simulink library "NREL5MW_Library"  (Simulink 8.2)
settings: Solver=ode45  StartTime=0.0  StopTime=10.0  RelTol=1e-3
undefined symbols (not defined in the file): NDOF, NumOuts, OutList, Parameter, q_init, qdot_init, strmatch, x1_t0
libraries: NREL5MW_Library x6, simulink x1
settings Model: Creator=raach  LastModifiedBy=schlipf

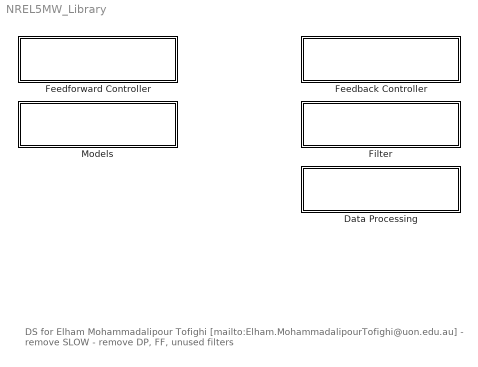
== system NREL5MW_Library ==
  note: DS for Elham Mohammadalipour Tofighi [mailto:Elham.MohammadalipourTofighi@uon.edu.au]
      | - remove SLOW
      | - remove DP, FF, unused filters
  Data Processing : Subsystem
      mask Display: fprintf('Data Processing')
  Feedback Controller : Subsystem
      mask Display: disp('Feedback Controller')
  Feedforward Controller : Subsystem
      mask Display: disp('Feedforward Controller')
  Filter : Subsystem
      mask Display: fprintf('Filter')
  Models : Subsystem
      mask Display: disp('Models')

== system NREL5MW_Library/Data Processing ==

== system NREL5MW_Library/Feedback Controller ==
  Feedback Controller : Subsystem
  Pitch Controller : Subsystem
  Torque Controller : Subsystem

== system NREL5MW_Library/Feedforward Controller ==

== system NREL5MW_Library/Filter ==
  FilterGenSpeed : Subsystem
  FilterSwitchR3 : Subsystem

== system NREL5MW_Library/Models ==
  FAST : Subsystem
  Generator : Subsystem
  Pitch Actuator : Subsystem

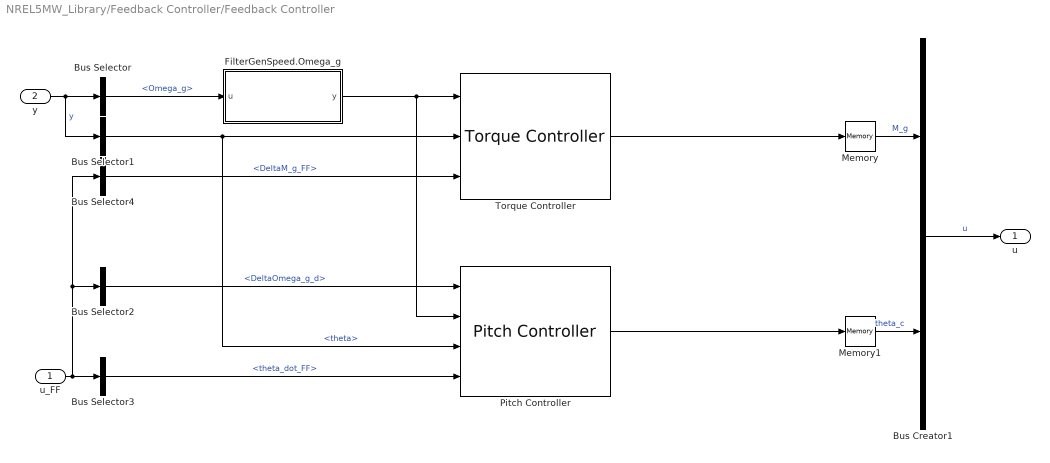
== system NREL5MW_Library/Feedback Controller/Feedback Controller ==
  u_FF : Inport
  y : Inport  Port=2
  Bus Creator1 : BusCreator  Inputs=2
  Bus Selector : BusSelector  OutputSignals=Omega_g
  Bus Selector1 : BusSelector  OutputSignals=theta
  Bus Selector2 : BusSelector  OutputSignals=DeltaOmega_g_d
  Bus Selector3 : BusSelector  OutputSignals=theta_dot_FF
  Bus Selector4 : BusSelector  OutputSignals=DeltaM_g_FF
  FilterGenSpeed.Omega_g : Subsystem
  Memory : Memory  X0=[Parameter.IC.M_g]
  Memory1 : Memory  X0=[Parameter.IC.theta]
  Pitch Controller : NREL5MW_Library/Feedback Controller/Pitch Controller
  Torque Controller : NREL5MW_Library/Feedback Controller/Torque Controller
  u : Outport
  wires:
  Bus Selector2/1 -> Pitch Controller/1  "<DeltaOmega_g_d>"
  Bus Selector/1 -> FilterGenSpeed.Omega_g/1(u)  "<Omega_g>"
  Bus Selector3/1 -> Pitch Controller/4  "<theta_dot_FF>"
  u_FF/1 -> Bus Selector3/1, Bus Selector4/1, Bus Selector2/1
  Pitch Controller/1 -> Memory1/1
  Bus Creator1/1 -> u/1  "u"
  Memory1/1 -> Bus Creator1/2  "theta_c"
  Memory/1 -> Bus Creator1/1  "M_g"
  Bus Selector1/1 -> Pitch Controller/3, Torque Controller/2  "<theta>"
  FilterGenSpeed.Omega_g/1(y) -> Torque Controller/1, Pitch Controller/2
  Torque Controller/1 -> Memory/1
  y/1 -> Bus Selector/1, Bus Selector1/1  "y"
  Bus Selector4/1 -> Torque Controller/3  "<DeltaM_g_FF>"

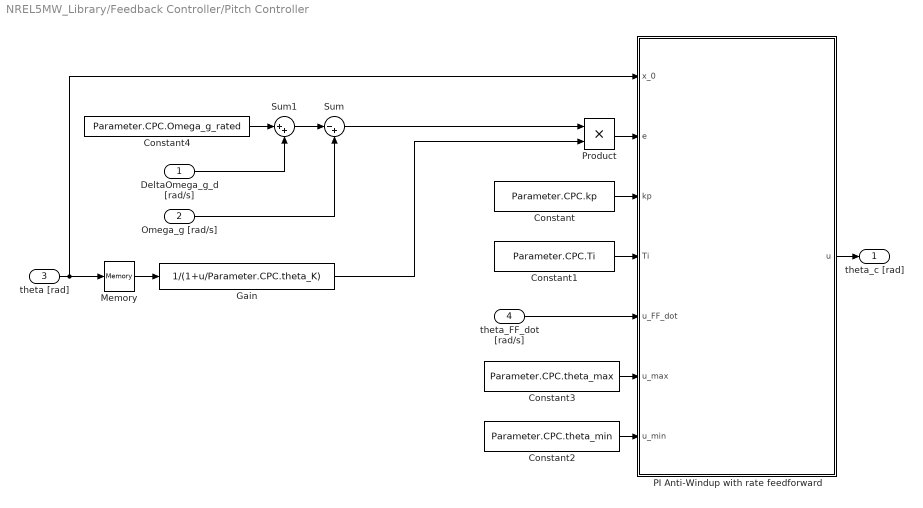
== system NREL5MW_Library/Feedback Controller/Pitch Controller ==
  DeltaOmega_g_d [rad/s] : Inport
  Omega_g [rad/s] : Inport  Port=2
  theta [rad] : Inport  Port=3
  theta_FF_dot [rad/s] : Inport  Port=4
  Constant : Constant  Value=Parameter.CPC.kp
  Constant1 : Constant  Value=Parameter.CPC.Ti
  Constant2 : Constant  Value=Parameter.CPC.theta_min
  Constant3 : Constant  Value=Parameter.CPC.theta_max
  Constant4 : Constant  Value=Parameter.CPC.Omega_g_rated
  Gain : Fcn  Expr=1/(1+u/Parameter.CPC.theta_K)
  Memory : Memory  X0=Parameter.IC.theta
  PI Anti-Windup with rate feedforward : Subsystem
  Product : Product  RndMeth=Zero
  Sum : Sum  Inputs=|-+
  Sum1 : Sum  Inputs=|++
  theta_c [rad] : Outport
  wires:
  Memory/1 -> Gain/1
  theta [rad]/1 -> PI Anti-Windup with rate feedforward/1(x_0), Memory/1
  Omega_g [rad/s]/1 -> Sum/2
  Gain/1 -> Product/2
  Sum/1 -> Product/1
  Product/1 -> PI Anti-Windup with rate feedforward/2(e)
  theta_FF_dot [rad/s]/1 -> PI Anti-Windup with rate feedforward/5(u_FF_dot)
  PI Anti-Windup with rate feedforward/1(u) -> theta_c [rad]/1
  Constant/1 -> PI Anti-Windup with rate feedforward/3(kp)
  Constant1/1 -> PI Anti-Windup with rate feedforward/4(Ti)
  Constant2/1 -> PI Anti-Windup with rate feedforward/7(u_min)
  Constant3/1 -> PI Anti-Windup with rate feedforward/6(u_max)
  DeltaOmega_g_d [rad/s]/1 -> Sum1/2
  Sum1/1 -> Sum/1
  Constant4/1 -> Sum1/1

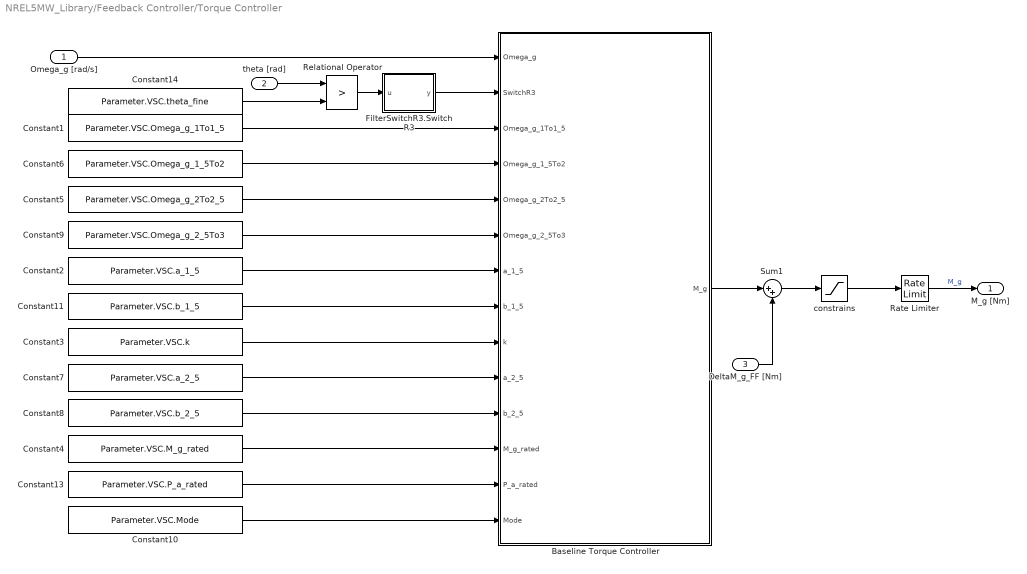
== system NREL5MW_Library/Feedback Controller/Torque Controller ==
  Omega_g [rad/s] : Inport
  theta [rad] : Inport  Port=2
  DeltaM_g_FF [Nm] : Inport  Port=3
  Baseline Torque Controller : MATLAB Function  TreatAsAtomicUnit=on
  Constant1 : Constant  Value=Parameter.VSC.Omega_g_1To1_5
  Constant10 : Constant  Value=Parameter.VSC.Mode
  Constant11 : Constant  Value=Parameter.VSC.b_1_5
  Constant13 : Constant  Value=Parameter.VSC.P_a_rated
  Constant14 : Constant  Value=Parameter.VSC.theta_fine
  Constant2 : Constant  Value=Parameter.VSC.a_1_5
  Constant3 : Constant  Value=Parameter.VSC.k
  Constant4 : Constant  Value=Parameter.VSC.M_g_rated
  Constant5 : Constant  Value=Parameter.VSC.Omega_g_2To2_5
  Constant6 : Constant  Value=Parameter.VSC.Omega_g_1_5To2
  Constant7 : Constant  Value=Parameter.VSC.a_2_5
  Constant8 : Constant  Value=Parameter.VSC.b_2_5
  Constant9 : Constant  Value=Parameter.VSC.Omega_g_2_5To3
  FilterSwitchR3.SwitchR3 : Subsystem
  Rate Limiter : RateLimiter  RisingSlewLimit=Parameter.VSC.M_g_dot_max  FallingSlewLimit=-Parameter.VSC.M_g_dot_max  SampleTimeMode=inherited  InitialCondition=Parameter.IC.M_g
  Relational Operator : RelationalOperator  Operator=>  OutDataTypeStr=boolean
  Sum1 : Sum  Inputs=|++
  constrains : Saturate  UpperLimit=Parameter.VSC.M_g_max  LowerLimit=Parameter.VSC.M_g_min
  M_g [Nm] : Outport
  wires:
  constrains/1 -> Rate Limiter/1
  Constant13/1 -> Baseline Torque Controller/13(P_a_rated)
  Constant11/1 -> Baseline Torque Controller/8(b_1_5)
  Constant2/1 -> Baseline Torque Controller/7(a_1_5)
  Constant10/1 -> Baseline Torque Controller/14(Mode)
  Constant3/1 -> Baseline Torque Controller/9(k)
  Constant7/1 -> Baseline Torque Controller/10(a_2_5)
  Constant8/1 -> Baseline Torque Controller/11(b_2_5)
  Constant4/1 -> Baseline Torque Controller/12(M_g_rated)
  Constant9/1 -> Baseline Torque Controller/6(Omega_g_2_5To3)
  Constant6/1 -> Baseline Torque Controller/4(Omega_g_1_5To2)
  Constant5/1 -> Baseline Torque Controller/5(Omega_g_2To2_5)
  Constant1/1 -> Baseline Torque Controller/3(Omega_g_1To1_5)
  Rate Limiter/1 -> M_g [Nm]/1  "M_g"
  Omega_g [rad/s]/1 -> Baseline Torque Controller/1(Omega_g)
  Baseline Torque Controller/1(M_g) -> Sum1/1
  Sum1/1 -> constrains/1
  DeltaM_g_FF [Nm]/1 -> Sum1/2
  Constant14/1 -> Relational Operator/2
  Relational Operator/1 -> FilterSwitchR3.SwitchR3/1(u)
  theta [rad]/1 -> Relational Operator/1
  FilterSwitchR3.SwitchR3/1(y) -> Baseline Torque Controller/2(SwitchR3)

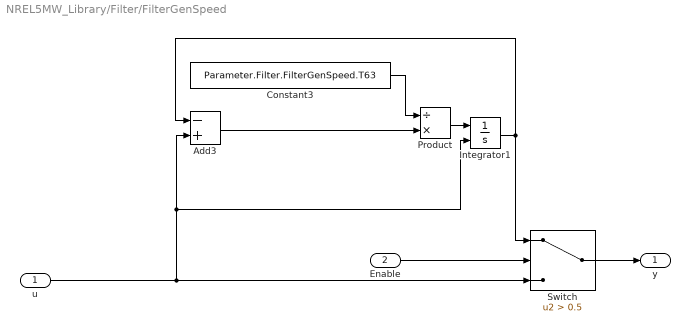
== system NREL5MW_Library/Filter/FilterGenSpeed ==
  u : Inport
  Enable : Inport  Port=2
  Add3 : Sum  Inputs=-+
  Constant3 : Constant  Value=Parameter.Filter.FilterGenSpeed.T63
  Integrator1 : Integrator  InitialConditionSource=external  InitialCondition=x1_t0
  Product : Product  Inputs=/*  RndMeth=Zero
  Switch : Switch  Criteria=u2 > Threshold  Threshold=0.5
  y : Outport
  wires:
  Constant3/1 -> Product/1
  Integrator1/1 -> Add3/1, Switch/1
  Product/1 -> Integrator1/1
  Add3/1 -> Product/2
  u/1 -> Switch/3, Integrator1/2, Add3/2
  Switch/1 -> y/1
  Enable/1 -> Switch/2

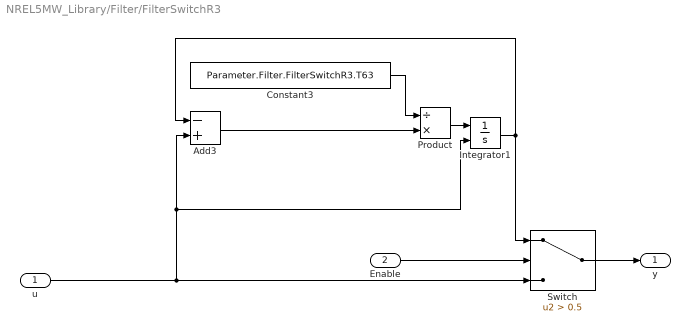
== system NREL5MW_Library/Filter/FilterSwitchR3 ==
  u : Inport
  Enable : Inport  Port=2
  Add3 : Sum  Inputs=-+
  Constant3 : Constant  Value=Parameter.Filter.FilterSwitchR3.T63
  Integrator1 : Integrator  InitialConditionSource=external  InitialCondition=x1_t0
  Product : Product  Inputs=/*  RndMeth=Zero
  Switch : Switch  Criteria=u2 > Threshold  Threshold=0.5
  y : Outport
  wires:
  Enable/1 -> Switch/2
  Switch/1 -> y/1
  u/1 -> Add3/2, Integrator1/2, Switch/3
  Add3/1 -> Product/2
  Product/1 -> Integrator1/1
  Integrator1/1 -> Switch/1, Add3/1
  Constant3/1 -> Product/1

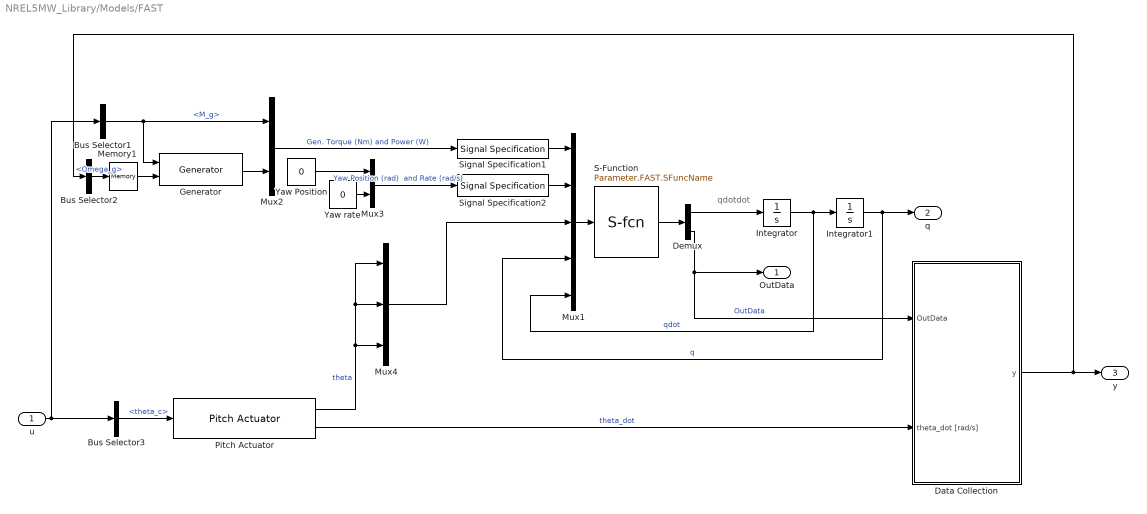
== system NREL5MW_Library/Models/FAST ==
  note: qdotdot
  u : Inport
  Bus Selector1 : BusSelector  OutputSignals=M_g
  Bus Selector2 : BusSelector  OutputSignals=Omega_g
  Bus Selector3 : BusSelector  OutputSignals=theta_c
  Data Collection : Subsystem
  Demux : Demux  Outputs=[NDOF, NumOuts]
  Generator : NREL5MW_Library/Models/Generator
  Integrator : Integrator  InitialCondition=qdot_init
  Integrator1 : Integrator  InitialCondition=q_init
  Memory1 : Memory  X0=Parameter.IC.Omega_g
  Mux1 : Mux  Inputs=5
  Mux2 : Mux  Inputs=2
  Mux3 : Mux  Inputs=2
  Mux4 : Mux  Inputs=3
  Pitch Actuator : NREL5MW_Library/Models/Pitch Actuator
  S-Function : S-Function  FunctionName=Parameter.FAST.SFuncName  EnableBusSupport=off
  Signal Specification1 : SignalSpecification  OutDataTypeStr=double  Dimensions=2
  Signal Specification2 : SignalSpecification  OutDataTypeStr=double  Dimensions=2
  Yaw Position : Constant  Value=0
  Yaw rate : Constant  Value=0
  OutData : Outport
  q : Outport  Port=2
  y : Outport  Port=3
  wires:
  Bus Selector1/1 -> Mux2/1, Generator/1  "<M_g>"
  Bus Selector3/1 -> Pitch Actuator/1  "<theta_c>"
  Pitch Actuator/2 -> Data Collection/2(theta_dot [rad/s])  "theta_dot"
  Mux4/1 -> Mux1/3
  u/1 -> Bus Selector3/1, Bus Selector1/1
  Integrator/1 -> Integrator1/1, Mux1/5  "qdot"
  Mux2/1 -> Signal Specification1/1  "Gen. Torque (Nm) and Power (W)"
  S-Function/1 -> Demux/1
  Demux/1 -> Integrator/1
  Demux/2 -> Data Collection/1(OutData), OutData/1  "OutData"
  Mux1/1 -> S-Function/1
  Mux3/1 -> Signal Specification2/1  "Yaw Position (rad)  and Rate (rad/s)"
  Integrator1/1 -> q/1, Mux1/4  "q"
  Signal Specification1/1 -> Mux1/1
  Signal Specification2/1 -> Mux1/2
  Yaw Position/1 -> Mux3/1
  Yaw rate/1 -> Mux3/2
  Pitch Actuator/1 -> Mux4/3, Mux4/1, Mux4/2  "theta"
  Data Collection/1(y) -> y/1, Bus Selector2/1
  Memory1/1 -> Generator/2
  Bus Selector2/1 -> Memory1/1  "<Omega_g>"
  Generator/1 -> Mux2/2

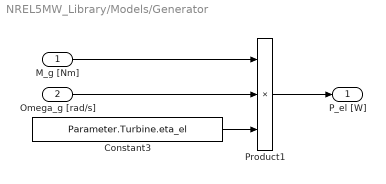
== system NREL5MW_Library/Models/Generator ==
  M_g [Nm] : Inport
  Omega_g [rad/s] : Inport  Port=2
  Constant3 : Constant  Value=Parameter.Turbine.eta_el
  Product1 : Product  Inputs=***  RndMeth=Zero
  P_el [W] : Outport
  wires:
  Constant3/1 -> Product1/3
  M_g [Nm]/1 -> Product1/1
  Product1/1 -> P_el [W]/1
  Omega_g [rad/s]/1 -> Product1/2

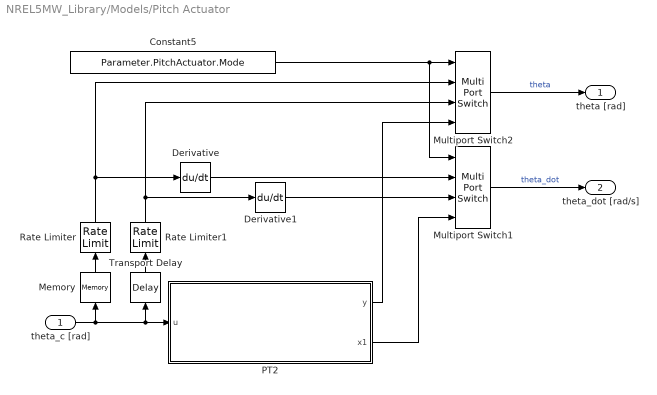
== system NREL5MW_Library/Models/Pitch Actuator ==
  theta_c [rad] : Inport
  Constant5 : Constant  Value=Parameter.PitchActuator.Mode
  Derivative : Derivative
  Derivative1 : Derivative
  Memory : Memory  X0=Parameter.IC.theta
  Multiport Switch1 : MultiPortSwitch  DataPortOrder=Specify indices  DataPortIndices={0,1,2}
  Multiport Switch2 : MultiPortSwitch  DataPortOrder=Specify indices  DataPortIndices={0,1,2}
  PT2 : Subsystem  mask{omega=Parameter.PitchActuator.omega, xi=Parameter.PitchActuator.xi, x1_t0=0, x2_t0=Parameter.IC.theta, x1_con=Parameter.PitchActuator.theta_dot_max, x2_max=Parameter.PitchActuator.theta_max, x2_min=Parameter.PitchActuator.theta_min}
      mask prompts: omega "undamped natural frequency [rad/s]"; xi "damping factor [-]"; x1_t0 "Inicial condition first state"; x2_t0 "Inicial condition second state"; x1_con "Constraint on first state (abs(x1)<=x1_con)"; x2_max "Upper bound x2"; x2_min "Lower bound x2"
      mask Display:
      | disp(['omega = ',num2str(omega),'\n'...
      |     ,'xi = ',num2str(xi),'\n'...
      |     ,'x1(t0) = ',num2str(x1_t0),'\n'...
      |     ,'x2(t0) = ',num2str(x2_t0),'\n'...
      |     ,'abs(x1) <= ',num2str(x1_con)])
      | port_label('output',1,'y')
      | port_label('output',2,'x1')
      | port_label('input',1,'u')
  Rate Limiter : RateLimiter  RisingSlewLimit=Parameter.PitchActuator.theta_dot_max  FallingSlewLimit=-Parameter.PitchActuator.theta_dot_max  SampleTimeMode=inherited  InitialCondition=Parameter.IC.theta
  Rate Limiter1 : RateLimiter  RisingSlewLimit=Parameter.PitchActuator.theta_dot_max  FallingSlewLimit=-Parameter.PitchActuator.theta_dot_max  SampleTimeMode=inherited  InitialCondition=Parameter.IC.theta
  Transport Delay : TransportDelay  DelayTime=Parameter.PitchActuator.Delay  InitialOutput=Parameter.IC.theta
  theta [rad] : Outport
  theta_dot [rad/s] : Outport  Port=2
  wires:
  Memory/1 -> Rate Limiter/1
  Rate Limiter/1 -> Multiport Switch2/2, Derivative/1
  Multiport Switch1/1 -> theta_dot [rad/s]/1  "theta_dot"
  Derivative/1 -> Multiport Switch1/2
  Multiport Switch2/1 -> theta [rad]/1  "theta"
  theta_c [rad]/1 -> Memory/1, Transport Delay/1, PT2/1(u)
  Constant5/1 -> Multiport Switch1/1, Multiport Switch2/1
  PT2/1(y) -> Multiport Switch2/4
  PT2/2(x1) -> Multiport Switch1/4
  Derivative1/1 -> Multiport Switch1/3
  Transport Delay/1 -> Rate Limiter1/1
  Rate Limiter1/1 -> Derivative1/1, Multiport Switch2/3

== system NREL5MW_Library/Feedback Controller/Feedback Controller/FilterGenSpeed.Omega_g ==
  u : Inport
  Constant3 : Constant  Value=Parameter.Filter.FilterGenSpeed.Omega_g.Enable
  FilterGenSpeed : NREL5MW_Library/Filter/FilterGenSpeed
  y : Outport
  wires:
  FilterGenSpeed/1 -> y/1
  u/1 -> FilterGenSpeed/1
  Constant3/1 -> FilterGenSpeed/2

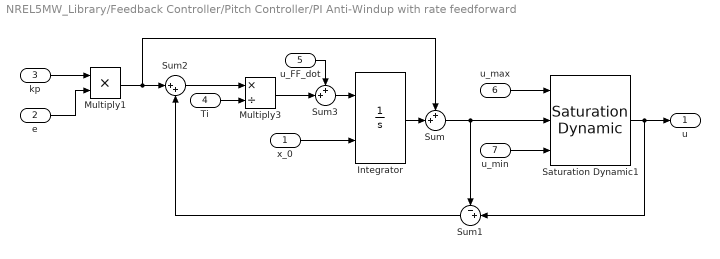
== system NREL5MW_Library/Feedback Controller/Pitch Controller/PI Anti-Windup with rate feedforward ==
  x_0 : Inport
  e : Inport  Port=2
  kp : Inport  Port=3
  Ti : Inport  Port=4
  u_FF_dot : Inport  Port=5
  u_max : Inport  Port=6
  u_min : Inport  Port=7
  Integrator : Integrator  InitialConditionSource=external
  Multiply1 : Product  Inputs=**
  Multiply3 : Product  Inputs=*/
  Saturation Dynamic1 : simulink/Discontinuities/Saturation Dynamic  OutMin=[]  OutMax=[]  OutDataTypeStr=Inherit: Same as second input  OutDataType=fixdt(1, 16)  OutScaling=2^-10  DoSatur=off
  Sum : Sum  Inputs=++|
  Sum1 : Sum  Inputs=-+|
  Sum2 : Sum  Inputs=|++
  Sum3 : Sum  Inputs=++|
  u : Outport
  wires:
  Saturation Dynamic1/1 -> u/1, Sum1/2
  Integrator/1 -> Sum/2
  kp/1 -> Multiply1/1
  e/1 -> Multiply1/2
  Ti/1 -> Multiply3/2
  Sum1/1 -> Sum2/2
  Multiply1/1 -> Sum/1, Sum2/1
  Sum2/1 -> Multiply3/1
  x_0/1 -> Integrator/2
  Multiply3/1 -> Sum3/2
  Sum3/1 -> Integrator/1
  u_FF_dot/1 -> Sum3/1
  u_min/1 -> Saturation Dynamic1/3
  Sum/1 -> Saturation Dynamic1/2, Sum1/1
  u_max/1 -> Saturation Dynamic1/1

== system NREL5MW_Library/Feedback Controller/Torque Controller/FilterSwitchR3.SwitchR3 ==
  u : Inport
  Constant3 : Constant  Value=Parameter.Filter.FilterSwitchR3.SwitchR3.Enable
  Data Type Conversion : DataTypeConversion  OutDataTypeStr=double
  FilterSwitchR3 : NREL5MW_Library/Filter/FilterSwitchR3
  y : Outport
  wires:
  Constant3/1 -> FilterSwitchR3/2
  u/1 -> Data Type Conversion/1
  FilterSwitchR3/1 -> y/1
  Data Type Conversion/1 -> FilterSwitchR3/1

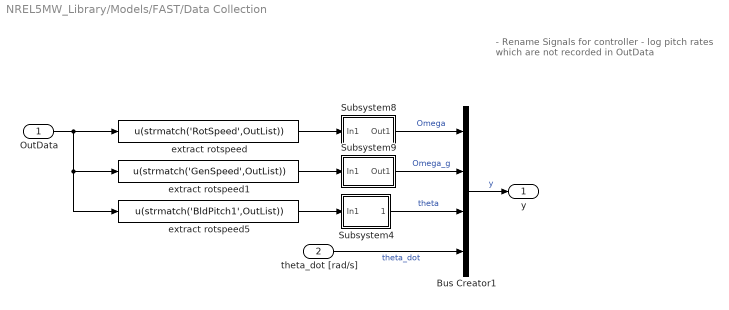
== system NREL5MW_Library/Models/FAST/Data Collection ==
  note: - Rename Signals for controller
      | - log pitch rates which are not recorded in OutData
  OutData : Inport
  theta_dot [rad/s] : Inport  Port=2
  Bus Creator1 : BusCreator
  Subsystem4 : Subsystem
      mask Display: disp('deg2rad')
  Subsystem8 : Subsystem
      mask Display: disp('rpm2rad/s')
  Subsystem9 : Subsystem
      mask Display: disp('rpm2rad/s')
  extract rotspeed : Fcn  Expr=u(strmatch('RotSpeed',OutList))
  extract rotspeed1 : Fcn  Expr=u(strmatch('GenSpeed',OutList))
  extract rotspeed5 : Fcn  Expr=u(strmatch('BldPitch1',OutList))
  y : Outport
  wires:
  Subsystem9/1(Out1) -> Bus Creator1/2  "Omega_g"
  Subsystem8/1(Out1) -> Bus Creator1/1  "Omega"
  extract rotspeed5/1 -> Subsystem4/1(In1)
  Bus Creator1/1 -> y/1  "y"
  extract rotspeed1/1 -> Subsystem9/1(In1)
  extract rotspeed/1 -> Subsystem8/1(In1)
  OutData/1 -> extract rotspeed1/1, extract rotspeed5/1, extract rotspeed/1
  Subsystem4/1(Out1) -> Bus Creator1/3  "theta"
  theta_dot [rad/s]/1 -> Bus Creator1/4  "theta_dot"

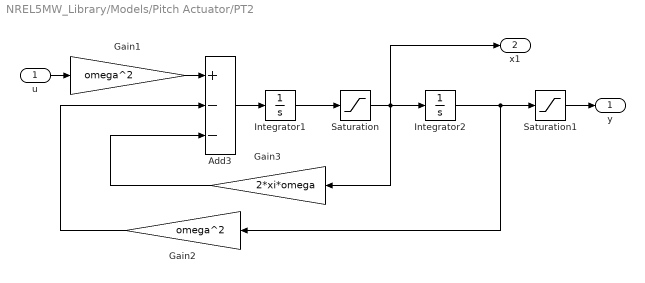
== system NREL5MW_Library/Models/Pitch Actuator/PT2 ==
  u : Inport
  Add3 : Sum  Inputs=+--
  Gain1 : Gain  Gain=omega^2  SaturateOnIntegerOverflow=on  OutDataTypeStr=Inherit: Same as input  ParamDataTypeStr=Inherit: Same as input
  Gain2 : Gain  Gain=omega^2  SaturateOnIntegerOverflow=on  OutDataTypeStr=Inherit: Same as input  ParamDataTypeStr=Inherit: Same as input
  Gain3 : Gain  Gain=2*xi*omega  SaturateOnIntegerOverflow=on  OutDataTypeStr=Inherit: Same as input  ParamDataTypeStr=Inherit: Same as input
  Integrator1 : Integrator  InitialCondition=x1_t0
  Integrator2 : Integrator  InitialCondition=x2_t0
  Saturation : Saturate  UpperLimit=x1_con  LowerLimit=-x1_con
  Saturation1 : Saturate  UpperLimit=x2_max  LowerLimit=x2_min
  y : Outport
  x1 : Outport  Port=2
  wires:
  Saturation1/1 -> y/1
  Gain3/1 -> Add3/3
  Integrator2/1 -> Saturation1/1, Gain2/1
  Integrator1/1 -> Saturation/1
  u/1 -> Gain1/1
  Add3/1 -> Integrator1/1
  Gain1/1 -> Add3/1
  Gain2/1 -> Add3/2
  Saturation/1 -> x1/1, Gain3/1, Integrator2/1

== system NREL5MW_Library/Models/FAST/Data Collection/Subsystem4 ==
  In1 : Inport
  deg in rad : Gain  Gain=2*pi/360  SaturateOnIntegerOverflow=on  OutDataTypeStr=Inherit: Same as input  ParamDataTypeStr=Inherit: Same as input
  Out1 : Outport
  wires:
  In1/1 -> deg in rad/1
  deg in rad/1 -> Out1/1

== system NREL5MW_Library/Models/FAST/Data Collection/Subsystem8 ==
  In1 : Inport
  rpm in rad/s : Gain  Gain=2*pi/60  SaturateOnIntegerOverflow=on  OutDataTypeStr=Inherit: Same as input  ParamDataTypeStr=Inherit: Same as input
  Out1 : Outport
  wires:
  rpm in rad/s/1 -> Out1/1
  In1/1 -> rpm in rad/s/1

== system NREL5MW_Library/Models/FAST/Data Collection/Subsystem9 ==
  In1 : Inport
  rpm in rad/s : Gain  Gain=2*pi/60  SaturateOnIntegerOverflow=on  OutDataTypeStr=Inherit: Same as input  ParamDataTypeStr=Inherit: Same as input
  Out1 : Outport
  wires:
  In1/1 -> rpm in rad/s/1
  rpm in rad/s/1 -> Out1/1

== matlab function Feedback Controller/Torque Controller/Baseline Torque Controller ==
  settings: fimath=|
      | fimath(...
      | 'RoundMode', 'floor',...
      | 'OverflowMode', 'wrap',...
      | 'ProductMode', 'KeepLSB', 'ProductWordLength', 32,...
      | 'SumMode', 'KeepLSB', 'SumWordLength', 32,...
      | 'CastBeforeSum', false)
  data: Omega_g input double; SwitchR3 input double; Omega_g_1To1_5 input double; Omega_g_1_5To2 input double; Omega_g_2To2_5 input double; Omega_g_2_5To3 input double; a_1_5 input double; b_1_5 input double; k input double; a_2_5 input double; b_2_5 input double; M_g output double; M_g_rated input double; P_a_rated input double; Mode input double
function M_g = BaselineVSControl(Omega_g,SwitchR3,...                          % signals
    Omega_g_1To1_5,Omega_g_1_5To2,Omega_g_2To2_5,Omega_g_2_5To3,...         % region limits
    a_1_5,b_1_5,...                         % Region 1.5 parameters
    k,...                                   % Region   2 parameters
    a_2_5,b_2_5,...                         % Region 2.5 parameters
    M_g_rated,P_a_rated,Mode)    % Region   3 parameters

if  Mode == 1   % Power constant
    M_g_3 = P_a_rated/Omega_g;
else            % Torque constant
    M_g_3 = M_g_rated;
end

if      Omega_g_2_5To3  <   Omega_g     % Region 3
    M_g     = M_g_3;

elseif  Omega_g_2To2_5  <   Omega_g     % Region 2.5
    M_g_2_5 = a_2_5 * Omega_g + b_2_5;
    M_g     = SwitchR3*M_g_3+(1-SwitchR3)*M_g_2_5;

elseif  Omega_g_1_5To2  <   Omega_g     % Region 2
    M_g_2   = k * Omega_g^2;
    M_g     = SwitchR3*M_g_3+(1-SwitchR3)*M_g_2;  
    
elseif  Omega_g_1To1_5  <   Omega_g     % Region 1.5
    M_g = a_1_5 * Omega_g + b_1_5;

else                                    % Region 1 
    M_g = 0;    
end
